simulink model "untitled3"  (R2024b)
settings: Solver=VariableStepAuto  StartTime=0.0  StopTime=200  RelTol=1e-3
values from neighbouring files (symbols this model uses):
  R = 0.246    [Ex_6.m]
undefined symbols (not defined in the file or in its folder): denC, denG, numC, numG
settings Model: Creator=EdoPolito  LastModifiedBy=EdoPolito

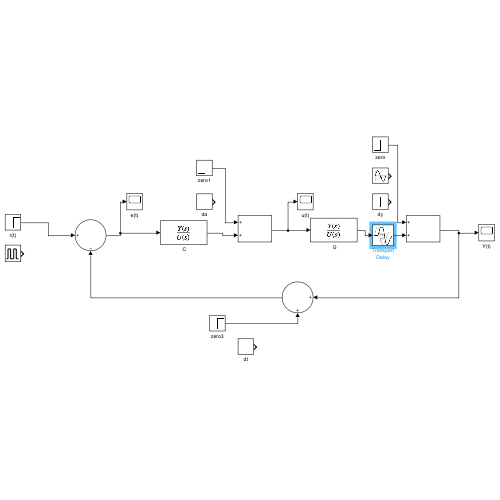
[thumbnail: Simulink's stored preview of the top-level diagram]
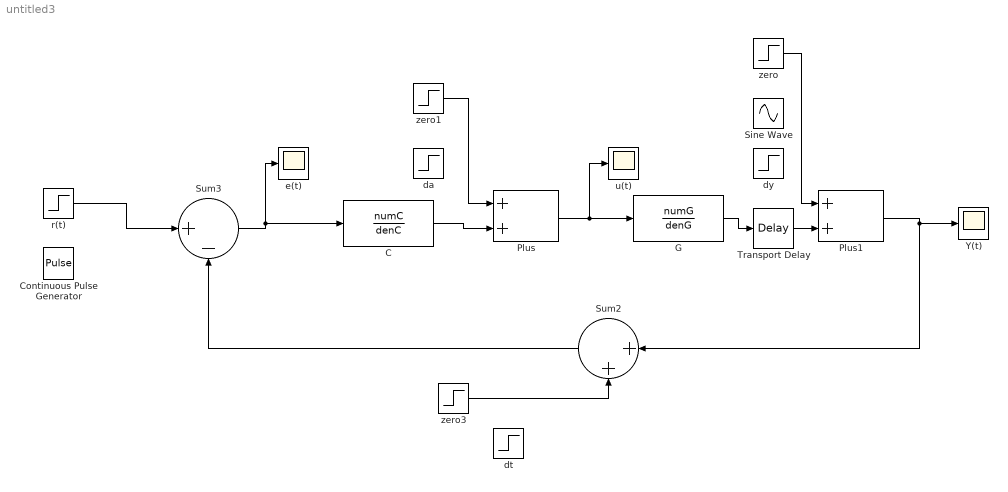
== system untitled3 ==
  " C" : TransferFcn  Numerator=numC  Denominator=denC
  " G" : TransferFcn  Numerator=numG  Denominator=denG
  Continuous Pulse Generator : DiscretePulseGenerator  PulseType=Time based  Period=1  PulseWidth=50
  Plus : Sum
  Plus1 : Sum
  Sine Wave : Sin  Amplitude=0.5  SampleTime=0
  Sum2 : Sum  Inputs=|++
  Sum3 : Sum  Inputs=|+-
  Transport Delay : TransportDelay  DelayTime=R
  Y(t) : Scope
  da : Step  Time=0  After=0  SampleTime=0
  dt : Step  Time=0  After=0  SampleTime=0
  dy : Step  Time=0  After=2  SampleTime=0
  e(t) : Scope
  r(t) : Step  Time=0  SampleTime=0
  u(t) : Scope
  zero : Step  Time=0  After=0  SampleTime=0
  zero1 : Step  Time=0  After=0  SampleTime=0
  zero3 : Step  Time=0  After=0  SampleTime=0
  wires:
  Plus1/1 -> Y(t)/1, Sum2/1
  Sum3/1 -> " C"/1, e(t)/1
  " C"/1 -> Plus/2
  zero1/1 -> Plus/1
  Sum2/1 -> Sum3/2
  Plus/1 -> u(t)/1, " G"/1
  zero3/1 -> Sum2/2
  zero/1 -> Plus1/1
  r(t)/1 -> Sum3/1
  Transport Delay/1 -> Plus1/2
  " G"/1 -> Transport Delay/1
